simulink model "inhneuronv1"  (Simulink 7.6)
settings: Solver=ode45  StartTime=0.0  StopTime=10.0  RelTol=1e-3
values from neighbouring files (symbols this model uses):
  amp = 1    [excneuroninit.m]
  neurodist = 1    [excneuroninit.m]
  sigslope = 3    [excneuroninit.m]
  tau_v = 0.1    [excneuroninit.m]
libraries: simulink x2
settings Model: Creator=root  LastModifiedBy=root

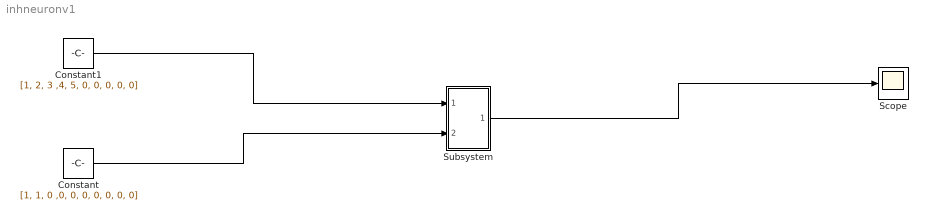
== system inhneuronv1 ==
  Constant : Constant  Value=[1, 1, 0 ,0, 0, 0, 0, 0, 0, 0]
  Constant1 : Constant  Value=[1, 2, 3 ,4, 5, 0, 0, 0, 0, 0]
  Scope : Scope
  Subsystem : Subsystem
  wires:
  Constant1/1 -> Subsystem/1(In2)
  Subsystem/1(Out2) -> Scope/1
  Constant/1 -> Subsystem/2(In1)

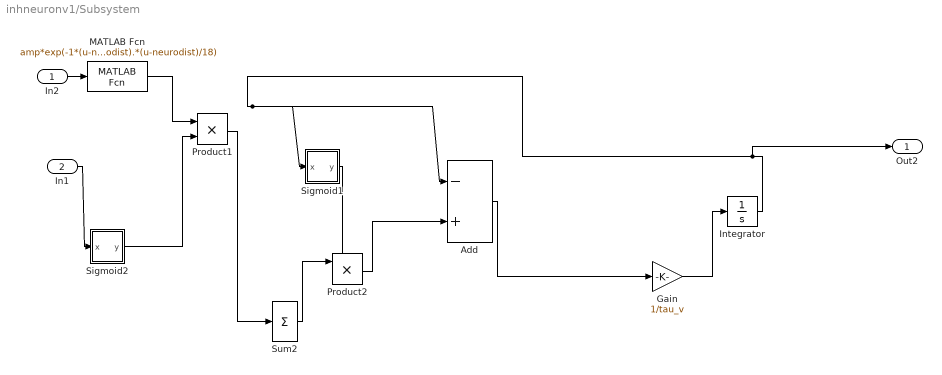
== system inhneuronv1/Subsystem ==
  In2 : Inport
  In1 : Inport  Port=2
  Add : Sum  Inputs=-+
  Gain : Gain  Gain=1/tau_v
  Integrator : Integrator  InitialCondition=1
  MATLAB Fcn : MATLABFcn  MATLABFcn=amp*exp(-1*(u-neurodist).*(u-neurodist)/18)  OutputDimensions=maxcon
  Product1 : Product  RndMeth=Zero
  Product2 : Product  RndMeth=Zero
  Sigmoid1 : Subsystem  TreatAsAtomicUnit=on  mask{slope=sigslope, offset=0.5}
      mask help: Created by Han, Cheol
      mask Display: plot([10 15 20 25 30 35 40 45 50], [0 0.01 0.1 0.2 0.5 0.8 0.9 0.99 1])
  Sigmoid2 : Subsystem  TreatAsAtomicUnit=on  mask{slope=sigslope, offset=0.5}
      mask help: Created by Han, Cheol
      mask Display: plot([10 15 20 25 30 35 40 45 50], [0 0.01 0.1 0.2 0.5 0.8 0.9 0.99 1])
  Sum2 : Sum  Inputs=+  SaturateOnIntegerOverflow=on
  Out2 : Outport
  wires:
  Add/1 -> Gain/1
  Gain/1 -> Integrator/1
  Integrator/1 -> Add/1, Sigmoid1/1(x), Out2/1
  MATLAB Fcn/1 -> Product1/1
  Sigmoid2/1(y) -> Product1/2
  Product1/1 -> Sum2/1
  Sum2/1 -> Product2/1
  Sigmoid1/1(y) -> Product2/2
  In2/1 -> MATLAB Fcn/1
  In1/1 -> Sigmoid2/1(x)
  Product2/1 -> Add/2

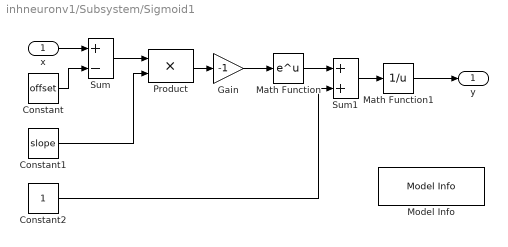
== system inhneuronv1/Subsystem/Sigmoid1 ==
  x : Inport
  Constant : Constant  Value=offset
  Constant1 : Constant  Value=slope
  Constant2 : Constant
  Gain : Gain  Gain=-1  SaturateOnIntegerOverflow=on  OutDataTypeStr=Inherit: Same as input  ParamDataTypeStr=Inherit: Same as input
  Math Function : Math  SaturateOnIntegerOverflow=on
  Math Function1 : Math  Operator=reciprocal  SaturateOnIntegerOverflow=on
  Model Info : simulink/Model-Wide Utilities/Model Info  SystemSampleTime=-1  InitialBlockCM=None  BlockCM=None  Frame=on  DisplayStringWithTags=|  HorizontalTextAlignment=Center  LeftAlignmentValue=0.5  SourceBlockDiagram=inhneuronv1  TagMaxNumber=20
      | Model Info
      | %<Creator> Han, Cheol
  Product : Product  SaturateOnIntegerOverflow=on  OutDataTypeStr=Inherit: Same as first input
  Sum : Sum  Inputs=+-  SaturateOnIntegerOverflow=on
  Sum1 : Sum  SaturateOnIntegerOverflow=on
  y : Outport  InitialOutput=0
  wires:
  x/1 -> Sum/1
  Constant/1 -> Sum/2
  Sum/1 -> Product/1
  Constant1/1 -> Product/2
  Product/1 -> Gain/1
  Gain/1 -> Math Function/1
  Math Function/1 -> Sum1/1
  Constant2/1 -> Sum1/2
  Sum1/1 -> Math Function1/1
  Math Function1/1 -> y/1

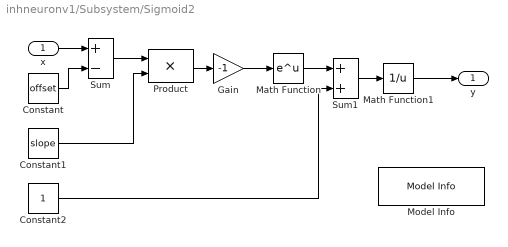
== system inhneuronv1/Subsystem/Sigmoid2 ==
  x : Inport
  Constant : Constant  Value=offset
  Constant1 : Constant  Value=slope
  Constant2 : Constant
  Gain : Gain  Gain=-1  SaturateOnIntegerOverflow=on  OutDataTypeStr=Inherit: Same as input  ParamDataTypeStr=Inherit: Same as input
  Math Function : Math  SaturateOnIntegerOverflow=on
  Math Function1 : Math  Operator=reciprocal  SaturateOnIntegerOverflow=on
  Model Info : simulink/Model-Wide Utilities/Model Info  SystemSampleTime=-1  InitialBlockCM=None  BlockCM=None  Frame=on  DisplayStringWithTags=|  HorizontalTextAlignment=Center  LeftAlignmentValue=0.5  SourceBlockDiagram=inhneuronv1  TagMaxNumber=20
      | Model Info
      | %<Creator> Han, Cheol
  Product : Product  SaturateOnIntegerOverflow=on  OutDataTypeStr=Inherit: Same as first input
  Sum : Sum  Inputs=+-  SaturateOnIntegerOverflow=on
  Sum1 : Sum  SaturateOnIntegerOverflow=on
  y : Outport  InitialOutput=0
  wires:
  x/1 -> Sum/1
  Constant/1 -> Sum/2
  Sum/1 -> Product/1
  Constant1/1 -> Product/2
  Product/1 -> Gain/1
  Gain/1 -> Math Function/1
  Math Function/1 -> Sum1/1
  Constant2/1 -> Sum1/2
  Sum1/1 -> Math Function1/1
  Math Function1/1 -> y/1
